simulink model "CL_Plant"  (R2017a)
settings: Solver=VariableStepAuto  StartTime=0.0  StopTime=450  RelTol=1e-3
values from neighbouring files (symbols this model uses):
  A_new = zeros(6,6)    [main_1.m]
  B_new = zeros(6,2)    [main_1.m]
  C_new = [1 0 0 0 0 0;0 1 0 0 0 0;0 0 1 0 0 0]    [main_1.m]
  D_new = zeros(3,2)    [main_1.m]
libraries: cstblocks x1
settings Model: Creator=Ali  LastModifiedBy=Ali

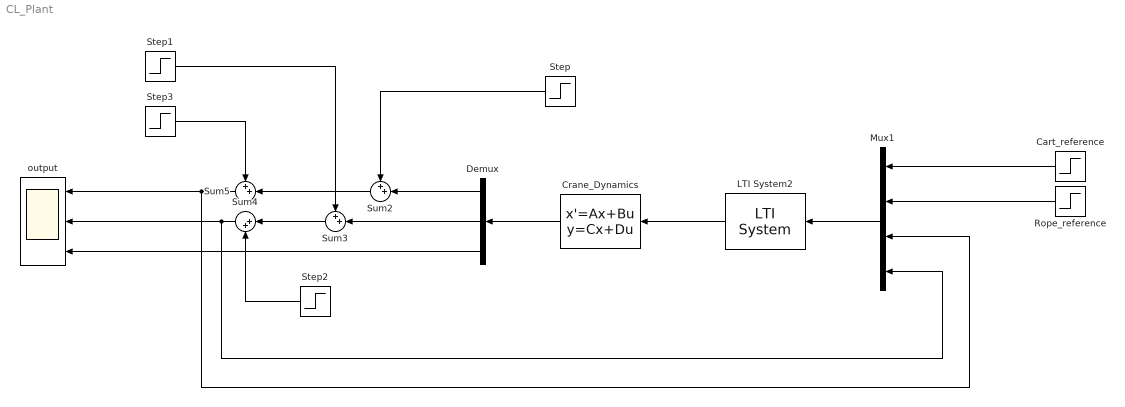
== system CL_Plant ==
  Cart_reference : Step  After=5  SampleTime=0
  Crane_Dynamics : StateSpace  A=A_new  B=B_new  C=C_new  D=D_new  X0=0
  Demux : Demux  Outputs=3
  LTI System2 : cstblocks/LTI System  sys=Kmu2  IC=[]
  Mux1 : Mux
  Rope_reference : Step  After=2  SampleTime=0
  Step : Step  Time=20  After=5  SampleTime=0
  Step1 : Step  Time=10  After=-8  SampleTime=0
  Step2 : Step  Time=5  After=10  SampleTime=0
  Step3 : Step  Time=35  After=15  SampleTime=0
  Sum2 : Sum  Inputs=++|
  Sum3 : Sum  Inputs=++|
  Sum4 : Sum  Inputs=|++
  Sum5 : Sum  Inputs=++|
  output : Scope  NumInputPorts=3
  wires:
  Mux1/1 -> LTI System2/1
  Demux/3 -> output/3
  Rope_reference/1 -> Mux1/2
  Sum4/1 -> output/2, Mux1/4
  Cart_reference/1 -> Mux1/1
  Step3/1 -> Sum5/1
  Demux/1 -> Sum2/2
  Sum2/1 -> Sum5/2
  Crane_Dynamics/1 -> Demux/1
  Demux/2 -> Sum3/2
  Sum3/1 -> Sum4/1
  Step2/1 -> Sum4/2
  Step1/1 -> Sum3/1
  LTI System2/1 -> Crane_Dynamics/1
  Step/1 -> Sum2/1
  Sum5/1 -> output/1, Mux1/3
